simulink model "p5p5e"  (Simulink 9.2)
settings: Solver=ode45  StartTime=0.0  StopTime=3000  RelTol=1e-3  EnableMultiTasking=on
values from neighbouring files (symbols this model uses):
  K_pd = 0.707    [p5p5c_init.m]    (also in p5p5d_init.m; p5p5e_init.m; p5p5f_init.m = 0.8406)
  reference = 30    [p5p5c_init.m]    (also in p5p5d_init.m; p5p5e_init.m = 0; p5p5f_init.m = 0)
  T_d = T    (= 71.3716)    [p5p5c_init.m]    (also in p5p5d_init.m; p5p5e_init.m; p5p5f_init.m)
  T_f = 10    [p5p5c_init.m]    (also in p5p5d_init.m; p5p5e_init.m; p5p5f_init.m = 8.391)
  T_s = 1/f_s    (= 0.1)    [p5p5c_init.m]    (also in p5p5d_init.m; p5p5e_init.m; p5p5f_init.m)
libraries: simulink x1
settings Model: Creator=markh  LastModifiedBy=Odin
settings DataIOCC: SignalLoggingName=sigsOut
settings OptimizationCC: InitFltsAndDblsToZero=on
settings DebuggingCC: SaveWithParameterizedLinksMsg=none  UnderspecifiedInitializationDetection=Simplified  SignalResolutionControl=TryResolveAllWithWarning  MultiTaskDSMMsg=warning  MultiTaskCondExecSysMsg=none
settings HardwareCC: TargetUnknown=on
settings GRTTargetCC: TargetFcnLib=ansi_tfl_tmw.mat

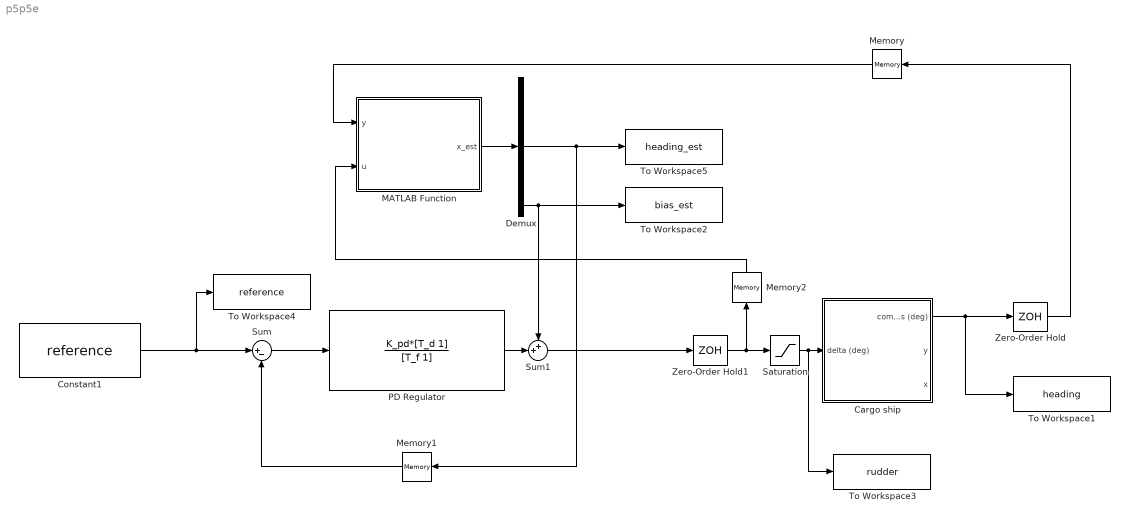
== system p5p5e ==
  Cargo ship : Subsystem  mask(Simple shipmodel for a cargo ship){noise=on, current=on, logic=on}
      mask prompts: noise "measurement noise"; logic "waves"
      mask help:
      | Measurement noise:
      | 	checked = noise on
      | 	unchecked = noise off
      |
      | Current:
      | 	checked = current on
      | 	unchecked = current off
      |
      | Waves:
      | 	checked = waves on
      | 	unchecked = waves off
      |
      | Author: Jørgen Spjøtvold, 9/10-2003
      | TTK 4115 Linear system theory.
      | Modified by Jostein Bakkeheim 26/10-2006
  Constant1 : Constant  Value=reference
  Demux : Demux  Outputs=5
  MATLAB Function : MATLAB Function  TreatAsAtomicUnit=on
  Memory : Memory
  Memory1 : Memory
  Memory2 : Memory
  PD Regulator : TransferFcn  Numerator=K_pd*[T_d 1]  Denominator=[T_f 1]
  Saturation : Saturate  UpperLimit=45  LowerLimit=-45
  Sum : Sum  Inputs=|+-
  Sum1 : Sum  Inputs=++|
  To Workspace1 : ToWorkspace  VariableName=heading  SaveFormat=Structure With Time  SampleTime=-1
  To Workspace2 : ToWorkspace  VariableName=bias_est  SaveFormat=Structure With Time  SampleTime=-1
  To Workspace3 : ToWorkspace  VariableName=rudder  SaveFormat=Structure With Time  SampleTime=-1
  To Workspace4 : ToWorkspace  VariableName=reference  SaveFormat=Structure With Time  SampleTime=-1
  To Workspace5 : ToWorkspace  VariableName=heading_est  SaveFormat=Structure With Time  SampleTime=-1
  Zero-Order Hold : ZeroOrderHold  SampleTime=T_s
  Zero-Order Hold1 : ZeroOrderHold  SampleTime=T_s
  wires:
  Cargo ship/1(compass (deg)) -> Zero-Order Hold/1, To Workspace1/1
  Constant1/1 -> To Workspace4/1, Sum/1
  Sum1/1 -> Zero-Order Hold1/1
  MATLAB Function/1(x_est) -> Demux/1
  Demux/5 -> Sum1/1, To Workspace2/1
  Zero-Order Hold/1 -> Memory/1
  PD Regulator/1 -> Sum1/2
  Sum/1 -> PD Regulator/1
  Zero-Order Hold1/1 -> Saturation/1, Memory2/1
  Saturation/1 -> To Workspace3/1, Cargo ship/1(delta (deg))
  Memory/1 -> MATLAB Function/1(y)
  Memory1/1 -> Sum/2
  Memory2/1 -> MATLAB Function/2(u)
  Demux/3 -> Memory1/1, To Workspace5/1

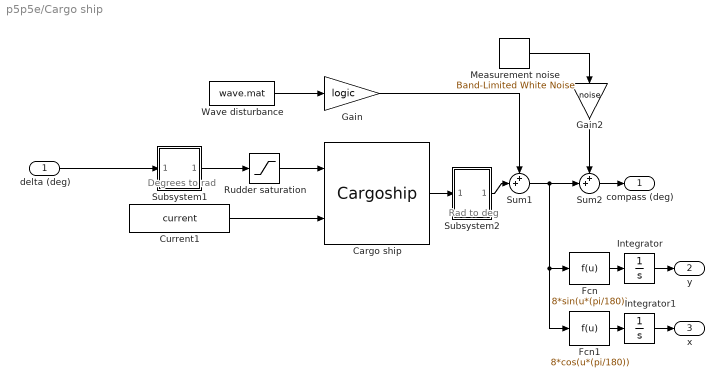
== system p5p5e/Cargo ship ==
  note: Degrees to rad
  note: Rad to deg
  delta (deg) : Inport
  Cargo ship : S-Function  FunctionName=Cargoship  SFunctionDeploymentMode=off  EnableBusSupport=off  mask(Cargo ship){}
      mask help:
      | S-function which simulates a cargo ship.
      |
      | Author: Jørgen Spjøtvold
      | 20.10-2003
      | Modified by Jostein Bakkeheim 27.10.2006
  Current1 : Constant  Value=current
  Fcn : Fcn  Expr=8*sin(u*(pi/180))
  Fcn1 : Fcn  Expr=8*cos(u*(pi/180))
  Gain : Gain  Gain=logic  SaturateOnIntegerOverflow=on  OutDataTypeStr=Inherit: Same as input  ParamDataTypeStr=Inherit: Same as input
  Gain2 : Gain  Gain=noise  SaturateOnIntegerOverflow=on  OutDataTypeStr=Inherit: Same as input  ParamDataTypeStr=Inherit: Same as input
  Integrator : Integrator
  Integrator1 : Integrator
  Measurement noise : simulink/Sources/Band-Limited White Noise  Cov=[0.001]  Ts=.5  seed=[23341]
  Rudder saturation : Saturate  UpperLimit=45*(pi/180)  LowerLimit=-45*(pi/180)
  Subsystem1 : Subsystem  mask(degrees to radians){}
      mask help: Converts degrees to radians
      mask Display: fprintf('D2R');
  Subsystem2 : Subsystem  mask(radians to degrees){}
      mask help: Converts radians to degrees
      mask Display: fprintf('R2D');
  Sum1 : Sum  Inputs=++|  SaturateOnIntegerOverflow=on
  Sum2 : Sum  Inputs=++|  SaturateOnIntegerOverflow=on
  Wave disturbance : FromFile  FileName=wave.mat  SampleTime=0
  compass (deg) : Outport
  y : Outport  Port=2
  x : Outport  Port=3
  wires:
  delta (deg)/1 -> Subsystem1/1(In1)
  Fcn/1 -> Integrator/1
  Integrator/1 -> y/1
  Fcn1/1 -> Integrator1/1
  Integrator1/1 -> x/1
  Wave disturbance/1 -> Gain/1
  Subsystem2/1(Out1) -> Sum1/2
  Gain/1 -> Sum1/1
  Sum1/1 -> Fcn/1, Fcn1/1, Sum2/2
  Cargo ship/1 -> Subsystem2/1(In1)
  Subsystem1/1(Out1) -> Rudder saturation/1
  Rudder saturation/1 -> Cargo ship/1
  Sum2/1 -> compass (deg)/1
  Measurement noise/1 -> Gain2/1
  Gain2/1 -> Sum2/1
  Current1/1 -> Cargo ship/2

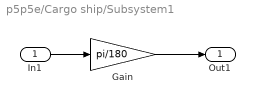
== system p5p5e/Cargo ship/Subsystem1 ==
  In1 : Inport
  Gain : Gain  Gain=pi/180  SaturateOnIntegerOverflow=on  OutDataTypeStr=Inherit: Same as input  ParamDataTypeStr=Inherit: Same as input
  Out1 : Outport
  wires:
  Gain/1 -> Out1/1
  In1/1 -> Gain/1

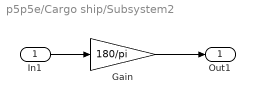
== system p5p5e/Cargo ship/Subsystem2 ==
  In1 : Inport
  Gain : Gain  Gain=180/pi  SaturateOnIntegerOverflow=on  OutDataTypeStr=Inherit: Same as input  ParamDataTypeStr=Inherit: Same as input
  Out1 : Outport
  wires:
  Gain/1 -> Out1/1
  In1/1 -> Gain/1

== matlab function MATLAB Function ==
  data: y input double; u input double; x_est output double; sys_init parameter Bus: slBus1
function x_est = kalman(y, u, sys_init)
    %% Declaring persistent variables    
    
    persistent x_est_ A B C E H Q R P_ init
    
    %% Initialisation
    if isempty(init)
       init    = 1;
        A      = sys_init.A_d;
        B      = sys_init.B_d;
        C      = sys_init.C_d;
        E      = sys_init.E_d;
        H      = sys_init.H_d;
        P_     = sys_init.P_0_;
        x_est_ = sys_init.x_est_0_;
        Q      = sys_init.Q;
        R      = sys_init.R;
        
    end
    
    %% Update y_est_
    
    y_est_ = C*x_est_;
    
    %% Calculate Kalman gain
    
    K = P_*C'*(C*P_*C' + H*R*H')^-1;
    
    %% Find a posteriori x_est
    
    x_est = x_est_ + K*(y - y_est_);
    
    %% Update covariance matrix P_

    P = P_ - K*C*P_ - P_*C'*K' + K*(C*P_*C' + H*R*H')*K';
    
    P_ = A*P*A' + E*Q*E';
    
    %% Update x_est_
    
    x_est_ = A*x_est + B*u;
end
